simulink model "Linear_observer"  (R2022a)
settings: Solver=VariableStepAuto  StartTime=0.0  StopTime=1000  RelTol=1e-3
values from neighbouring files (symbols this model uses):
  A = [0 0 0 ... (first row only)    [Lithium_ion_oneCell_Modeling_continuous_Linear.m]    (also in Lithium_ion_oneCell_Modeling_continuous_new.m)
  A_d = sys_d.A    [Lithium_ion_oneCell_Modeling_continuous_Linear.m]    (also in Lithium_ion_oneCell_Modeling_continuous_new.m)
  B = [-eta/C_max ... (first row only)    [Lithium_ion_oneCell_Modeling_continuous_Linear.m]    (also in Lithium_ion_oneCell_Modeling_continuous_new.m)
  B_d = sys_d.B    [Lithium_ion_oneCell_Modeling_continuous_Linear.m]    (also in Lithium_ion_oneCell_Modeling_continuous_new.m)
  bias = 3.551    [Lithium_ion_oneCell_Modeling_continuous_Linear.m]
  C = [0.5672 -1 -1]    [Lithium_ion_oneCell_Modeling_continuous_Linear.m]    (also in Lithium_ion_oneCell_Modeling_continuous_new.m = [0 -1 -1])
  C_d = sys_d.C    [Lithium_ion_oneCell_Modeling_continuous_Linear.m]
  D_d = sys_d.D    [Lithium_ion_oneCell_Modeling_continuous_Linear.m]
  L = acker(A_d',C_d',[0.001,0.001,0.001])'    [Lithium_ion_oneCell_Modeling_continuous_Linear.m]
  X0 = [0.6; 0; 0]    [Lithium_ion_oneCell_Modeling_continuous_Linear.m]    (also in Lithium_ion_oneCell_Modeling_continuous_new.m = [0.6;0;0])
libraries: simulink x1
settings Model: Creator=Asus  LastModifiedBy=Asus

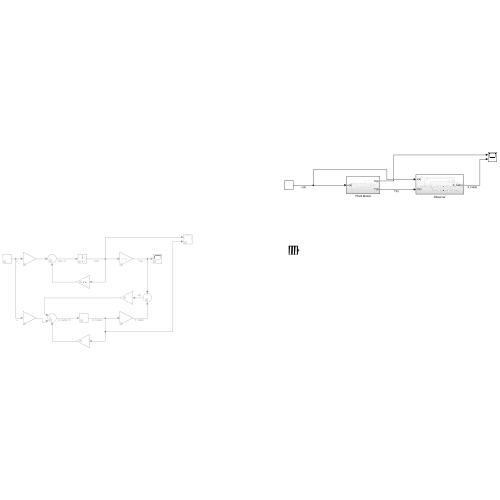
[thumbnail: Simulink's stored preview of the top-level diagram]
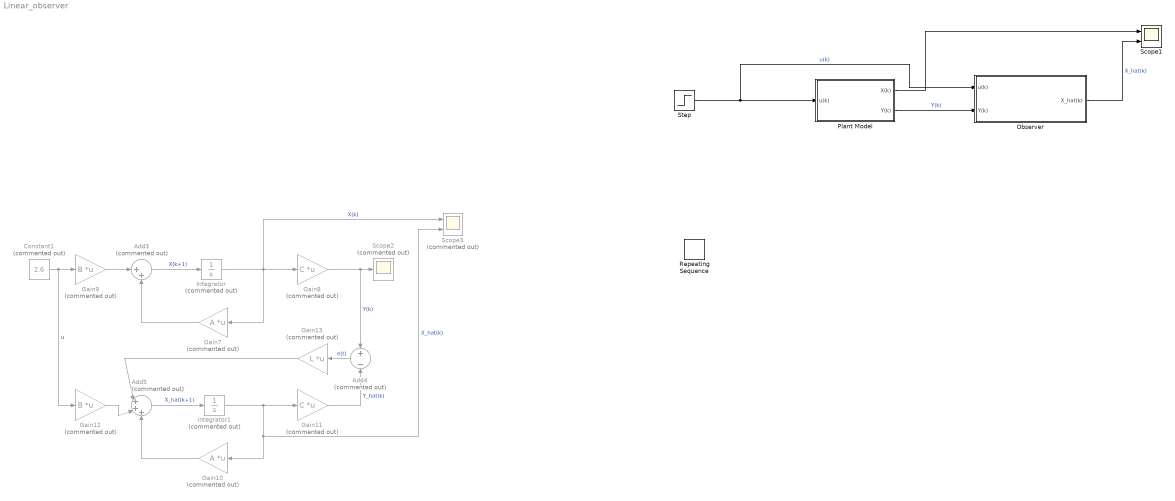
== system Linear_observer ==
  Add3 : Sum  Commented=on  Inputs=|++
  Add4 : Sum  Commented=on  Inputs=+-
  Add5 : Sum  Commented=on  Inputs=|+++
  Constant1 : Constant  Commented=on  Value=2.6
  Gain10 : Gain  Commented=on  Gain=A  Multiplication=Matrix(K*u)
  Gain11 : Gain  Commented=on  Gain=C  Multiplication=Matrix(K*u)
  Gain12 : Gain  Commented=on  Gain=B  Multiplication=Matrix(K*u)
  Gain13 : Gain  Commented=on  Gain=L  Multiplication=Matrix(K*u)
  Gain7 : Gain  Commented=on  Gain=A  Multiplication=Matrix(K*u)
  Gain8 : Gain  Commented=on  Gain=C  Multiplication=Matrix(K*u)
  Gain9 : Gain  Commented=on  Gain=B  Multiplication=Matrix(K*u)
  Integrator : Integrator  Commented=on  InitialCondition=X0
  Integrator1 : Integrator  Commented=on
  Observer : Subsystem
  Plant Model : Subsystem
  Repeating Sequence : simulink/Sources/Repeating Sequence  rep_seq_t=[0 2 4 6 8 10]  rep_seq_y=[0 2 2 2 2 2]
  Scope1 : Scope  NumInputPorts=2
  Scope2 : Scope  Commented=on
  Scope3 : Scope  Commented=on  NumInputPorts=2
  Step : Step  Time=10  Before=2.6  After=2.6  SampleTime=0
  wires:
  Step/1 -> Observer/1(u(k)), Plant Model/1(u(k))  "u(k)"
  Gain13/1 -> Add5/1
  Gain12/1 -> Add5/2
  Add5/1 -> Integrator1/1  "X_hat(k+1)"
  Add4/1 -> Gain13/1  "e(t)"
  Constant1/1 -> Gain12/1, Gain9/1  "u"
  Integrator1/1 -> Gain10/1, Scope3/2, Gain11/1  "X_hat(k)"
  Gain10/1 -> Add5/3
  Gain9/1 -> Add3/1
  Gain7/1 -> Add3/2
  Integrator/1 -> Scope3/1, Gain7/1, Gain8/1  "X(k)"
  Gain8/1 -> Add4/1, Scope2/1  "Y(k)"
  Gain11/1 -> Add4/2  "Y_hat(k)"
  Add3/1 -> Integrator/1  "X(k+1)"
  Plant Model/1(X(k)) -> Scope1/1
  Plant Model/2(Y(k)) -> Observer/2(Y(k))  "Y(k)"
  Observer/1(X_hat(k)) -> Scope1/2  "X_hat(k)"

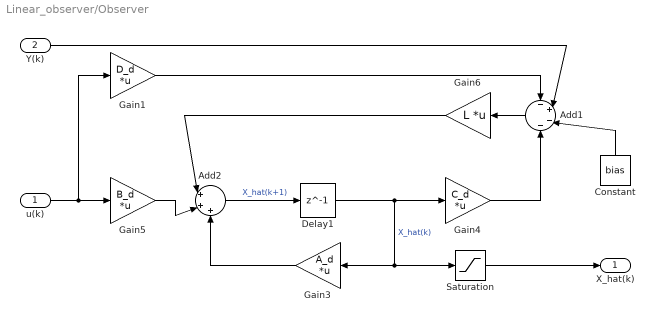
== system Linear_observer/Observer ==
  u(k) : Inport
  Y(k) : Inport  Port=2
  Add1 : Sum  Inputs=-+--
  Add2 : Sum  Inputs=|+++
  Constant : Constant  Value=bias
  Delay1 : Delay  DelayLength=1  InitialCondition=0
  Gain1 : Gain  Gain=D_d  Multiplication=Matrix(K*u)
  Gain3 : Gain  Gain=A_d  Multiplication=Matrix(K*u)
  Gain4 : Gain  Gain=C_d  Multiplication=Matrix(K*u)
  Gain5 : Gain  Gain=B_d  Multiplication=Matrix(K*u)
  Gain6 : Gain  Gain=L  Multiplication=Matrix(K*u)
  Saturation : Saturate  UpperLimit=[1;4.2;4.2]  LowerLimit=0
  X_hat(k) : Outport
  wires:
  Delay1/1 -> Gain3/1, Saturation/1, Gain4/1  "X_hat(k)"
  Add1/1 -> Gain6/1
  Gain5/1 -> Add2/2
  Gain3/1 -> Add2/3
  u(k)/1 -> Gain1/1, Gain5/1
  Gain6/1 -> Add2/1
  Add2/1 -> Delay1/1  "X_hat(k+1)"
  Y(k)/1 -> Add1/2
  Gain4/1 -> Add1/4
  Constant/1 -> Add1/3
  Gain1/1 -> Add1/1
  Saturation/1 -> X_hat(k)/1

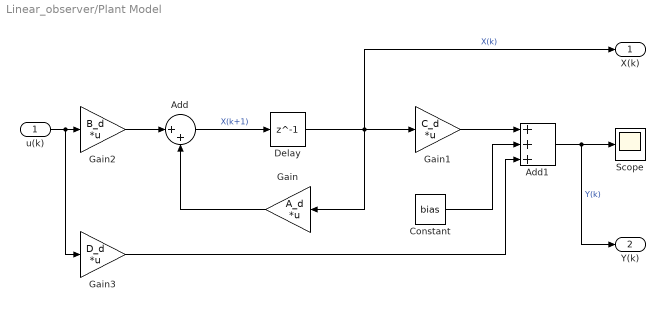
== system Linear_observer/Plant Model ==
  u(k) : Inport
  Add : Sum  Inputs=|++
  Add1 : Sum  Inputs=+++
  Constant : Constant  Value=bias
  Delay : Delay  DelayLength=1  InitialCondition=X0
  Gain : Gain  Gain=A_d  Multiplication=Matrix(K*u)
  Gain1 : Gain  Gain=C_d  Multiplication=Matrix(K*u)
  Gain2 : Gain  Gain=B_d  Multiplication=Matrix(K*u)
  Gain3 : Gain  Gain=D_d  Multiplication=Matrix(K*u)
  Scope : Scope
  X(k) : Outport
  Y(k) : Outport  Port=2
  wires:
  Delay/1 -> X(k)/1, Gain/1, Gain1/1  "X(k)"
  Gain/1 -> Add/2
  u(k)/1 -> Gain3/1, Gain2/1
  Add/1 -> Delay/1  "X(k+1)"
  Gain2/1 -> Add/1
  Gain1/1 -> Add1/1
  Constant/1 -> Add1/2
  Add1/1 -> Scope/1, Y(k)/1  "Y(k)"
  Gain3/1 -> Add1/3
